simulink model "test_mex_in_slx"  (R2024b)
settings: Solver=VariableStepAuto  StartTime=0.0  StopTime=10.0  RelTol=1e-3
settings Model: Creator=39340  LastModifiedBy=39340

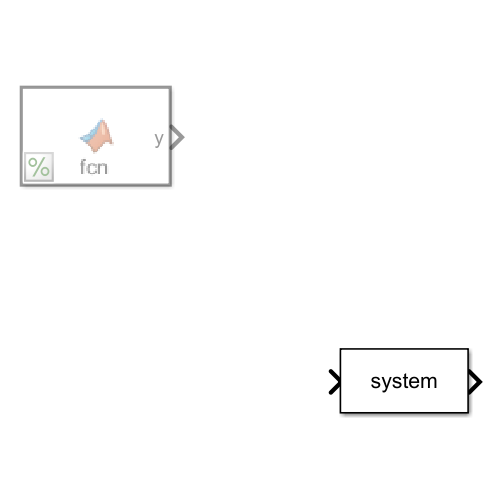
[thumbnail: Simulink's stored preview of the top-level diagram]
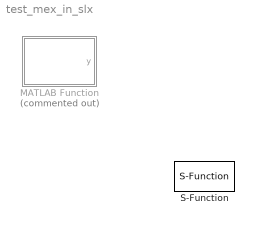
== system test_mex_in_slx ==
  MATLAB Function : MATLAB Function  Commented=on  TreatAsAtomicUnit=on
  S-Function : S-Function  SFunctionDeploymentMode=off  EnableBusSupport=off

== matlab function test_mex_in_slx/MATLAB Function ==
  data: y output
function y = fcn()

out = net_predict_L_40k_mex(rand(1,10,6));

y = out(1,end,1);
